simulink model "test_build_scan"  (Simulink 6.5)
settings: Solver=VariableStepDiscrete  StartTime=0.0  StopTime=10.0  RelTol=1e-3
libraries: xbsIndex_r4 x18, nort_sysgenlib x10
settings Model: Creator=nort  LastModifiedBy=nort

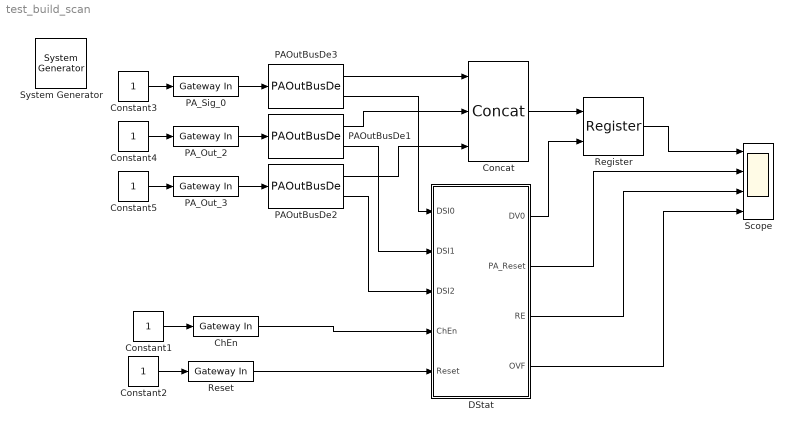
== system test_build_scan ==
  " System Generator" : xbsIndex_r4/ System Generator  Tag=genX  SystemSampleTime=-1  xilinxfamily=virtex4  part=xc4vlx25  speed=-10  package=ff668  synthesis_tool=XST  directory=./netlist  testbench=off  simulink_period=1  sysclk_period=10  incr_netlist=off  trim_vbits=Everywhere in SubSystem  dbl_ovrd=According to Block Masks  core_generation=According to Block Masks  run_coregen=off  deprecated_control=off  eval_field=0  block_type=sysgen
      settings: block_version=8.2
  ChEn : xbsIndex_r4/Gateway In  arith_type=Unsigned  n_bits=3  bin_pt=0  quantization="Round  (unbiased: +/- Inf)"  overflow=Wrap  period=1  dbl_ovrd=off  timing_constraint=Data Rate  locs_specified=off  LOCs={}  block_type=gatewayin
      settings: infoedit="Gateway in block.  Converts inputs of type Simulink integer, double and fixed point to  Xilinx fixed point type.<P><P>Hardware notes:  In hardware these blocks become top level input ports."
  Concat : xbsIndex_r4/Concat  num_inputs=3  dbl_ovrd=off  block_type=concat
      settings: block_version=9.2.01
  Constant{1..5} (5 alike) : Constant  Value=1  OutDataType=sfix(16)  ConRadixGroup=Use specified scaling  OutScaling=2^0  SampleTime=inf  FramePeriod=inf
  DStat : Subsystem
  PAOutBusDe1 : nort_sysgenlib/PAOutBusDe  SystemSampleTime=-1
  PAOutBusDe2 : nort_sysgenlib/PAOutBusDe  SystemSampleTime=-1
  PAOutBusDe3 : nort_sysgenlib/PAOutBusDe  SystemSampleTime=-1
  PA_Out_2 : xbsIndex_r4/Gateway In  arith_type=Unsigned  n_bits=28  bin_pt=0  quantization="Round  (unbiased: +/- Inf)"  overflow=Wrap  period=1  dbl_ovrd=off  timing_constraint=Data Rate  locs_specified=off  LOCs={}  block_type=gatewayin
      settings: infoedit="Gateway in block.  Converts inputs of type Simulink integer, double and fixed point to  Xilinx fixed point type.<P><P>Hardware notes:  In hardware these blocks become top level input ports."
  PA_Out_3 : xbsIndex_r4/Gateway In  arith_type=Unsigned  n_bits=28  bin_pt=0  quantization="Round  (unbiased: +/- Inf)"  overflow=Wrap  period=1  dbl_ovrd=off  timing_constraint=Data Rate  locs_specified=off  LOCs={}  block_type=gatewayin
      settings: infoedit="Gateway in block.  Converts inputs of type Simulink integer, double and fixed point to  Xilinx fixed point type.<P><P>Hardware notes:  In hardware these blocks become top level input ports."
  PA_Sig_0 : xbsIndex_r4/Gateway In  arith_type=Unsigned  n_bits=28  bin_pt=0  quantization="Round  (unbiased: +/- Inf)"  overflow=Wrap  period=1  dbl_ovrd=off  timing_constraint=Data Rate  locs_specified=off  LOCs={}  block_type=gatewayin
      settings: infoedit="Gateway in block.  Converts inputs of type Simulink integer, double and fixed point to  Xilinx fixed point type.<P><P>Hardware notes:  In hardware these blocks become top level input ports."
  Register : xbsIndex_r4/Register  init=0  rst=off  en=on  dbl_ovrd=off  block_type=register
      settings: block_version=9.2.01
  Reset : xbsIndex_r4/Gateway In  arith_type=Boolean  n_bits=1  bin_pt=0  quantization="Round  (unbiased: +/- Inf)"  overflow=Wrap  period=1  dbl_ovrd=off  timing_constraint=Data Rate  locs_specified=off  LOCs={}  block_type=gatewayin
      settings: infoedit="Gateway in block.  Converts inputs of type Simulink integer, double and fixed point to  Xilinx fixed point type.<P><P>Hardware notes:  In hardware these blocks become top level input ports."
  Scope : Scope  NumInputPorts=4
      settings: YMin=-5~-5~-5~-5  YMax=5~5~5~5
  wires:
  Constant3/1 -> PA_Sig_0/1
  Constant4/1 -> PA_Out_2/1
  Constant5/1 -> PA_Out_3/1
  PA_Out_2/1 -> PAOutBusDe1/1
  PA_Out_3/1 -> PAOutBusDe2/1
  Concat/1 -> Register/1
  PAOutBusDe1/1 -> Concat/2
  PAOutBusDe2/1 -> Concat/3
  PAOutBusDe1/2 -> DStat/2(DSI1)
  PAOutBusDe2/2 -> DStat/3(DSI2)
  DStat/1(DV0) -> Register/2
  Register/1 -> Scope/1
  DStat/2(PA_Reset) -> Scope/2
  DStat/3(RE) -> Scope/3
  DStat/4(OVF) -> Scope/4
  Constant1/1 -> ChEn/1
  ChEn/1 -> DStat/4(ChEn)
  Constant2/1 -> Reset/1
  Reset/1 -> DStat/5(Reset)
  PA_Sig_0/1 -> PAOutBusDe3/1
  PAOutBusDe3/1 -> Concat/1
  PAOutBusDe3/2 -> DStat/1(DSI0)

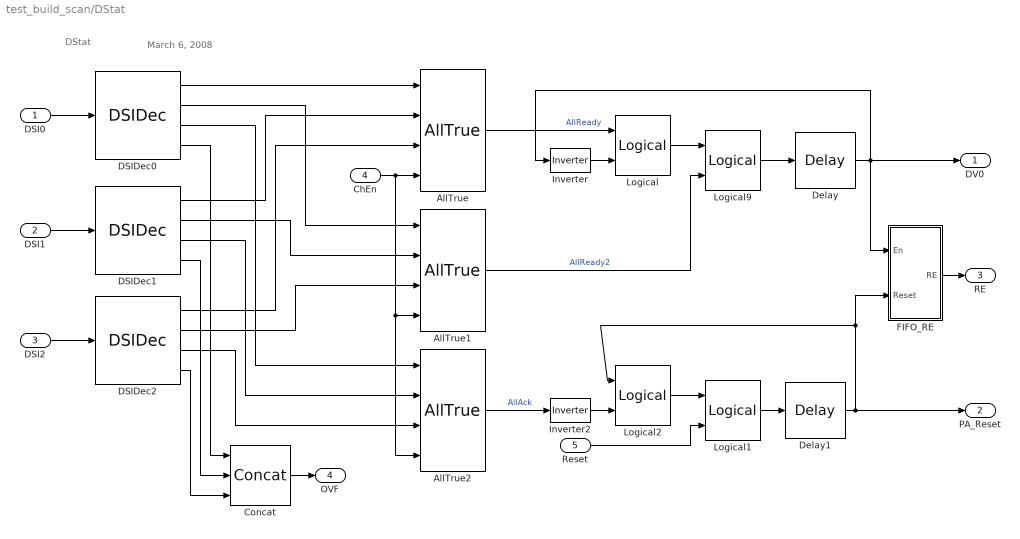
== system test_build_scan/DStat ==
  note: DStat
  note: March 6, 2008
  DSI0 : Inport
  DSI1 : Inport  Port=2
  DSI2 : Inport  Port=3
  ChEn : Inport  Port=4
  Reset : Inport  Port=5
  AllTrue : nort_sysgenlib/AllTrue  SystemSampleTime=-1
  AllTrue1 : nort_sysgenlib/AllTrue  SystemSampleTime=-1
  AllTrue2 : nort_sysgenlib/AllTrue  SystemSampleTime=-1
  Concat : xbsIndex_r4/Concat  num_inputs=3  dbl_ovrd=off  block_type=concat
      settings: block_version=9.2.01
  DSIDec0 : nort_sysgenlib/DSIDec  SystemSampleTime=-1
  DSIDec1 : nort_sysgenlib/DSIDec  SystemSampleTime=-1
  DSIDec2 : nort_sysgenlib/DSIDec  SystemSampleTime=-1
  Delay : xbsIndex_r4/Delay  en=off  latency=1  dbl_ovrd=off  reg_retiming=off  block_type=delay
      settings: block_version=9.2.01
  Delay1 : xbsIndex_r4/Delay  en=off  latency=1  dbl_ovrd=off  reg_retiming=off  block_type=delay
      settings: block_version=9.2.01
  FIFO_RE : Subsystem
  Inverter : xbsIndex_r4/Inverter  en=off  latency=0  dbl_ovrd=off  block_type=inv
      settings: block_version=9.2.01
  Inverter2 : xbsIndex_r4/Inverter  en=off  latency=0  dbl_ovrd=off  block_type=inv
      settings: block_version=9.2.01
  Logical : xbsIndex_r4/Logical  logical_function=AND  inputs=2  en=off  latency=0  precision=Full  arith_type=Unsigned  n_bits=16  bin_pt=0  align_bp=on  dbl_ovrd=off  block_type=logical
      settings: block_version=9.2.01
  Logical1 : xbsIndex_r4/Logical  logical_function=OR  inputs=2  en=off  latency=0  precision=Full  arith_type=Unsigned  n_bits=16  bin_pt=0  align_bp=on  dbl_ovrd=off  block_type=logical
      settings: block_version=9.2.01
  Logical2 : xbsIndex_r4/Logical  logical_function=AND  inputs=2  en=off  latency=0  precision=Full  arith_type=Unsigned  n_bits=16  bin_pt=0  align_bp=on  dbl_ovrd=off  block_type=logical
      settings: block_version=9.2.01
  Logical9 : xbsIndex_r4/Logical  logical_function=OR  inputs=2  en=off  latency=0  precision=Full  arith_type=Unsigned  n_bits=16  bin_pt=0  align_bp=on  dbl_ovrd=off  block_type=logical
      settings: block_version=9.2.01
  DV0 : Outport
  PA_Reset : Outport  Port=2
  RE : Outport  Port=3
  OVF : Outport  Port=4
  wires:
  DSIDec0/1 -> AllTrue/1
  DSIDec1/1 -> AllTrue/2
  DSIDec2/1 -> AllTrue/3
  AllTrue/1 -> Logical/1  "AllReady"
  Delay/1 -> DV0/1, Inverter/1, FIFO_RE/1(En)
  FIFO_RE/1(RE) -> RE/1
  DSI0/1 -> DSIDec0/1
  Inverter/1 -> Logical/2
  Logical/1 -> Logical9/1
  Logical9/1 -> Delay/1
  AllTrue1/1 -> Logical9/2  "AllReady2"
  DSI1/1 -> DSIDec1/1
  DSI2/1 -> DSIDec2/1
  DSIDec0/2 -> AllTrue1/1
  ChEn/1 -> AllTrue/4, AllTrue1/4, AllTrue2/4
  DSIDec1/2 -> AllTrue1/2
  DSIDec2/2 -> AllTrue1/3
  Reset/1 -> Logical1/2
  DSIDec0/3 -> AllTrue2/1
  DSIDec1/3 -> AllTrue2/2
  DSIDec2/3 -> AllTrue2/3
  AllTrue2/1 -> Inverter2/1  "AllAck"
  Logical2/1 -> Logical1/1
  Logical1/1 -> Delay1/1
  Inverter2/1 -> Logical2/2
  Delay1/1 -> PA_Reset/1, Logical2/1, FIFO_RE/2(Reset)
  DSIDec0/4 -> Concat/1
  DSIDec1/4 -> Concat/2
  DSIDec2/4 -> Concat/3
  Concat/1 -> OVF/1

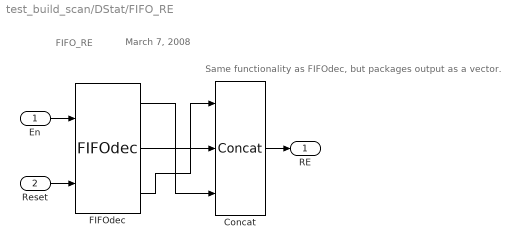
== system test_build_scan/DStat/FIFO_RE ==
  note: FIFO_RE
  note: March 7, 2008
  note: Same functionality as
      | FIFOdec, but packages
      | output as a vector.
  En : Inport
  Reset : Inport  Port=2
  Concat : xbsIndex_r4/Concat  num_inputs=3  dbl_ovrd=off  block_type=concat
      settings: block_version=9.2.01
  FIFOdec : nort_sysgenlib/FIFOdec  SystemSampleTime=-1
  RE : Outport
  wires:
  FIFOdec/1 -> Concat/3
  FIFOdec/2 -> Concat/2
  FIFOdec/3 -> Concat/1
  En/1 -> FIFOdec/1
  Concat/1 -> RE/1
  Reset/1 -> FIFOdec/2
